simulink model "CoagulationMPCSimulink"  (R2021a)
settings: Solver=VariableStepAuto  StartTime=0.0  StopTime=60  RelTol=1e-3
libraries: mpclib x2
settings Model: Creator=s.ghetmiri  LastModifiedBy=s.ghetmiri

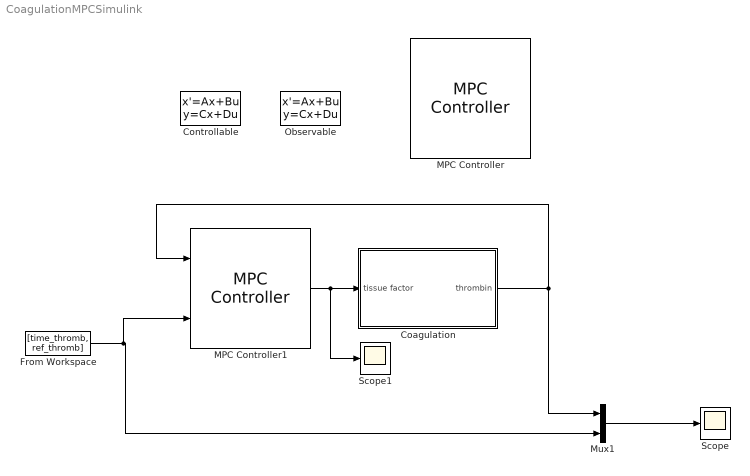
== system CoagulationMPCSimulink ==
  Coagulation : Subsystem
  Controllable : StateSpace  A=[0 1 0; 0 0 1; -0.5061 -2.3308 -2.126]  B=[0;0;1]  C=[1 0 0]  D=0  InitialCondition=0
  From Workspace : FromWorkspace  VariableName=[time_thromb, ref_thromb]  SampleTime=.5
  MPC Controller : mpclib/MPC Controller  SCDEnableBlockLinearizationSpecification=on  is_multiple=0  enable_value=0  return_u0=off  updateMPCinCallerWorkspace=on  md_inport=off  mv_inport=off  uref_inport=off  return_cost=off  return_mvseq=off  return_qpstatus=off  return_xseq=off  return_state=off  return_ovseq=off  state_inport=off  umin_inport=off  umax_inport=off  ymin_inport=off  ymax_inport=off  cc_inport=off  ywt_inport=off  uwt_inport=off  duwt_inport=off  rhoeps_inport=off  pm_inport=off  MaximumP=10  HorizonChoice=FixedHorizon  n_ts=0.5  n_p=10  n_mv=1  n_md=0  n_ud=0  n_mo=1  n_uo=0  BlockDataType=double  SampleTimeInherited=off  switch_inport=off
  MPC Controller1 : mpclib/MPC Controller  SCDEnableBlockLinearizationSpecification=on  is_multiple=0  enable_value=0  return_u0=off  updateMPCinCallerWorkspace=on  md_inport=off  mv_inport=off  uref_inport=off  return_cost=off  return_mvseq=off  return_qpstatus=off  return_xseq=off  return_state=off  return_ovseq=off  state_inport=off  umin_inport=off  umax_inport=off  ymin_inport=off  ymax_inport=off  cc_inport=off  ywt_inport=off  uwt_inport=off  duwt_inport=off  rhoeps_inport=off  pm_inport=off  MaximumP=10  HorizonChoice=FixedHorizon  n_ts=0.5  n_p=10  n_mv=1  n_md=1  n_ud=0  n_mo=1  n_uo=0  BlockDataType=double  SampleTimeInherited=off  switch_inport=off
  Mux1 : Mux  Inputs=2
  Observable : StateSpace  A=[-2.1261 1 0; -2.3308 0 1; -0.5061 0 0]  B=[0;0;2e5]  C=[1 0 0]  D=0  InitialCondition=0
  Scope : Scope
  Scope1 : Scope
  wires:
  From Workspace/1 -> MPC Controller1/2, Mux1/2
  Mux1/1 -> Scope/1
  Coagulation/1(thrombin) -> Mux1/1, MPC Controller1/1
  MPC Controller1/1 -> Scope1/1, Coagulation/1(tissue factor)

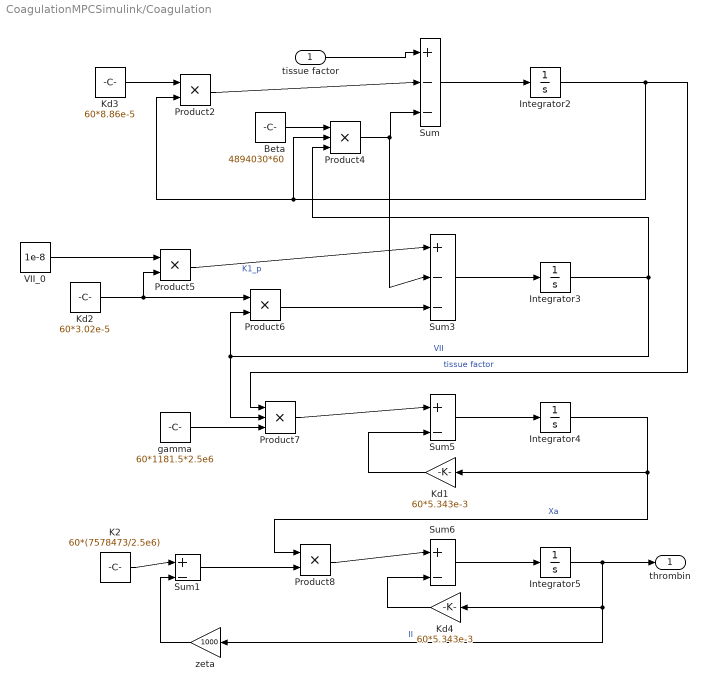
== system CoagulationMPCSimulink/Coagulation ==
  tissue factor : Inport
  Beta : Constant  Value=4894030*60
  Integrator2 : Integrator  InitialCondition=4.0056e-13  LimitOutput=on  LowerSaturationLimit=0
  Integrator3 : Integrator  InitialCondition=9.99999e-9  LimitOutput=on  LowerSaturationLimit=0
  Integrator4 : Integrator  InitialCondition=5.8328e-11  LimitOutput=on  LowerSaturationLimit=0
  Integrator5 : Integrator  InitialCondition=7.0411e-10  LimitOutput=on  LowerSaturationLimit=0
  K2 : Constant  Value=60*(7578473/2.5e6)
  Kd1 : Gain  Gain=60*5.343e-3
  Kd2 : Constant  Value=60*3.02e-5
  Kd3 : Constant  Value=60*8.86e-5
  Kd4 : Gain  Gain=60*5.343e-3
  Product{2,5..6,8} (4 alike) : Product
  Product4 : Product  Inputs=3
  Product7 : Product  Inputs=3
  Sum : Sum  Inputs=|+--
  Sum1 : Sum  Inputs=|+-
  Sum3 : Sum  Inputs=|+--
  Sum5 : Sum  Inputs=|+-
  Sum6 : Sum  Inputs=|+-
  VII_0 : Constant  Value=1e-8
  gamma : Constant  Value=60*1181.5*2.5e6
  zeta : Gain  Gain=1000
  thrombin : Outport
  wires:
  tissue factor/1 -> Sum/1
  Sum/1 -> Integrator2/1
  Integrator2/1 -> Product4/2, Product2/2, Product7/1  "tissue factor"
  Kd3/1 -> Product2/1
  Product2/1 -> Sum/2
  Beta/1 -> Product4/1
  Product4/1 -> Sum3/2, Sum/3
  Integrator3/1 -> Product7/2, Product6/2, Product4/3  "VII"
  Product5/1 -> Sum3/1  "K1_p"
  Sum3/1 -> Integrator3/1
  VII_0/1 -> Product5/1
  Kd2/1 -> Product5/2, Product6/1
  Product6/1 -> Sum3/3
  Sum5/1 -> Integrator4/1
  gamma/1 -> Product7/3
  Product7/1 -> Sum5/1
  Integrator4/1 -> Product8/1, Kd1/1  "Xa"
  Kd1/1 -> Sum5/2
  Sum6/1 -> Integrator5/1
  Integrator5/1 -> zeta/1, Kd4/1, thrombin/1  "II"
  Kd4/1 -> Sum6/2
  Product8/1 -> Sum6/1
  K2/1 -> Sum1/1
  zeta/1 -> Sum1/2
  Sum1/1 -> Product8/2
